simulink model "einfuehrung"  (R2023b)
settings: Solver=FixedStepAuto  StartTime=0.0  StopTime=10.0  FixedStep=0.01  RelTol=1e-3
libraries: simulink x1
settings Model: Creator=suttarar@hu-berlin.de  LastModifiedBy=suttarar@hu-berlin.de

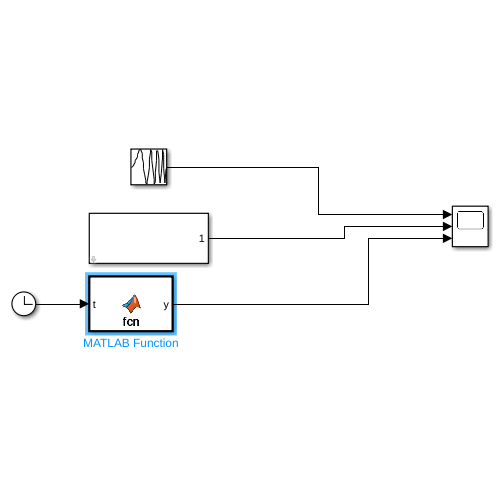
[thumbnail: Simulink's stored preview of the top-level diagram]
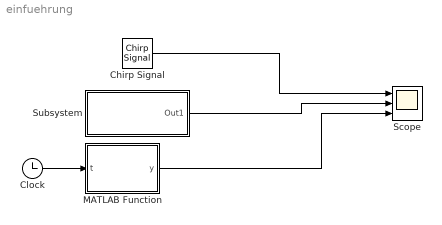
== system einfuehrung ==
  Chirp Signal : simulink/Sources/Chirp Signal  f1=0  T=10  f2=10
  Clock : Clock
  MATLAB Function : MATLAB Function  TreatAsAtomicUnit=on
  Scope : Scope  NumInputPorts=3
  Subsystem : Subsystem  mask{f0=0, f1=10, T=10}
      mask prompts: f0 "Startfrequenz"; f1 "Endfrequenz"; T "Dauer"
  wires:
  Subsystem/1(Out1) -> Scope/2
  Chirp Signal/1 -> Scope/1
  MATLAB Function/1(y) -> Scope/3
  Clock/1 -> MATLAB Function/1(t)

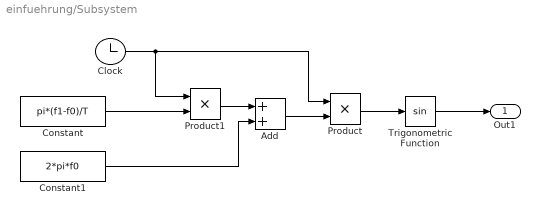
== system einfuehrung/Subsystem ==
  Add : Sum
  Clock : Clock
  Constant : Constant  Value=pi*(f1-f0)/T
  Constant1 : Constant  Value=2*pi*f0
  Product : Product
  Product1 : Product
  Trigonometric Function : Trigonometry
  Out1 : Outport
  wires:
  Trigonometric Function/1 -> Out1/1
  Product/1 -> Trigonometric Function/1
  Add/1 -> Product/2
  Product1/1 -> Add/1
  Clock/1 -> Product1/1, Product/1
  Constant1/1 -> Add/2
  Constant/1 -> Product1/2

== matlab function einfuehrung/MATLAB Function ==
  data: t input; y output
function y = fcn(t)

f0=0;
f1=10;
T=10;

k=(f1-f0)/T;
y = sin(pi.*t.*(2*f0+k.*t));
